simulink model "CompareToConstant_TestGen7"  (R2017b)
settings: Solver=FixedStepDiscrete  StartTime=0.0  StopTime=10.0  RelTol=1e-3
undefined symbols (not defined in the file): Block_TestLib, reset
libraries: simulink x1
settings Model: Creator=ktrinh  LastModifiedBy=ktrinh
settings DebuggingCC: ParameterOverflowMsg=none

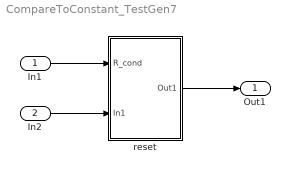
== system CompareToConstant_TestGen7 ==
  In1 : Inport
  In2 : Inport  Port=2
  reset : Subsystem  AncestorBlock=Block_TestLib/reset
  Out1 : Outport
  wires:
  In1/1 -> reset/1(R_cond)
  In2/1 -> reset/2(In1)
  reset/1(Out1) -> Out1/1

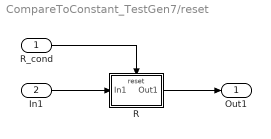
== system CompareToConstant_TestGen7/reset ==
  R_cond : Inport  OutDataTypeStr=boolean
  In1 : Inport  Port=2
  R : Subsystem  TreatAsAtomicUnit=on
  Out1 : Outport
  wires:
  R_cond/1 -> R/Reset
  In1/1 -> R/1(In1)
  R/1(Out1) -> Out1/1

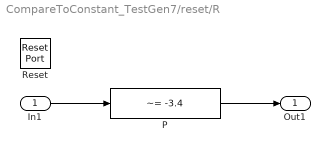
== system CompareToConstant_TestGen7/reset/R ==
  In1 : Inport  OutDataTypeStr=int32  PortDimensions=1
  Reset : ResetPort  DisableCoverage=on
  P : simulink/Logic and Bit Operations/Compare To Constant  relop=~=  const=-3.4  OutDataTypeStr=uint8
  Out1 : Outport
  wires:
  In1/1 -> P/1
  P/1 -> Out1/1
